simulink model "Analog_DSSS_WH"  (Simulink 7.5)
settings: Solver=ode45  SolverMode=SingleTasking  StartTime=0.0  StopTime=50  RelTol=1e-3
values from neighbouring files (symbols this model uses):
  Amp = Simulink.Parameter    [Analog_DSSS_GC_saveas.m]    (also in Analog_DSSS_WH_saveas.m)
  FreqBase = Simulink.Parameter    [Analog_DSSS_GC_saveas.m]    (also in Analog_DSSS_WH_saveas.m)
  Phs = Simulink.Parameter    [Analog_DSSS_GC_saveas.m]    (also in Analog_DSSS_WH_saveas.m)
libraries: dsparch4 x4, dspsnks4 x2
settings Model: Creator=rooki  LastModifiedBy=rooki  CovMetricSettings=dwe  CovHtmlReporting=off  covSaveCumulativeToWorkspaceVar=off  CovSaveSingleToWorkspaceVar=off  CovExternalEMLEnable=on
settings DataIOCC: LimitDataPoints=off  SaveFormat=StructureWithTime
settings OptimizationCC: ExpressionDepthLimit=128
settings DebuggingCC: UnderspecifiedInitializationDetection=Simplified  MergeDetectMultiDrivingBlocksExec=error  SolverPrmCheckMsg=none  FcnCallInpInsideContextMsg=Enable All  StateNameClashWarn=none
settings HardwareCC: ProdIntDivRoundTo=Zero  ProdEndianess=LittleEndian  ProdHWDeviceType=Specified
settings CodeAppCC: CustomSymbolStrType=$N$R$M_T
settings GRTTargetCC: TargetFunctionLibrary=C99 (ISO)  GeneratePreprocessorConditionals=Use local settings

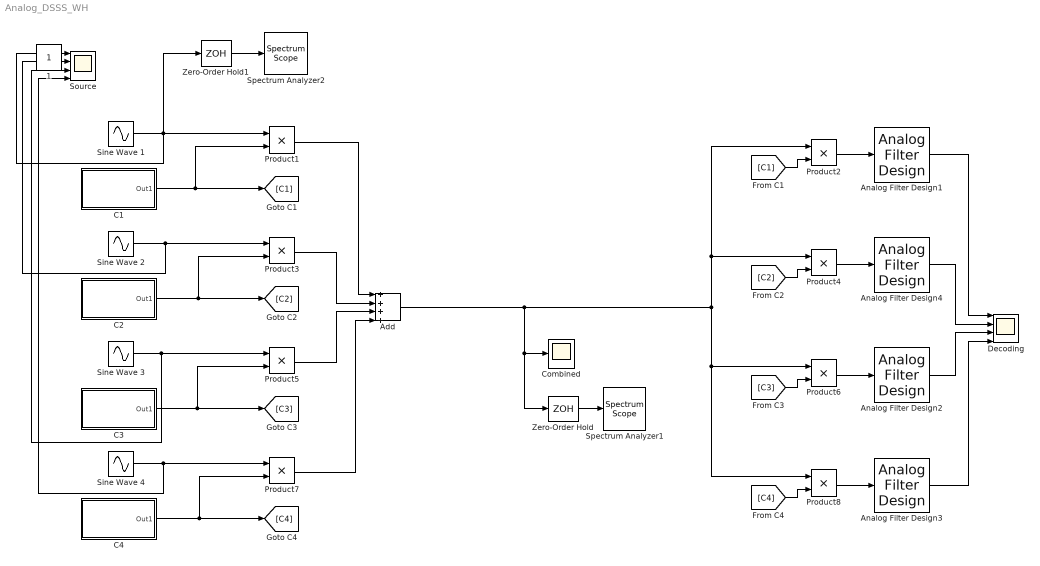
== system Analog_DSSS_WH ==
  Add : Sum  Inputs=++++
  Analog Filter Design{1..4} (4 alike) : dsparch4/Analog Filter Design  method=Butterworth  filttype=Lowpass  N=8  Wlo=2  Whi=80  Rp=2  Rs=40
  C1 : Subsystem  Description=Replaced Block
      mask Type: Replaced Block
      mask Description: This block has been replaced with an empty subsystem because it used functionality that is unavailable in Simulink R2010a.
      mask Display: fprintf('Replaced: %s\n','MATLABSystem')
  C2 : Subsystem  Description=Replaced Block
      mask Type: Replaced Block
      mask Description: This block has been replaced with an empty subsystem because it used functionality that is unavailable in Simulink R2010a.
      mask Display: fprintf('Replaced: %s\n','MATLABSystem')
  C3 : Subsystem  Description=Replaced Block
      mask Type: Replaced Block
      mask Description: This block has been replaced with an empty subsystem because it used functionality that is unavailable in Simulink R2010a.
      mask Display: fprintf('Replaced: %s\n','MATLABSystem')
  C4 : Subsystem  Description=Replaced Block
      mask Type: Replaced Block
      mask Description: This block has been replaced with an empty subsystem because it used functionality that is unavailable in Simulink R2010a.
      mask Display: fprintf('Replaced: %s\n','MATLABSystem')
  Combined : Scope
      settings: TimeRange=auto  MaxDataPoints=5000  SaveToWorkspace=off  SaveName=ScopeData2  YMin=-5.14393  YMax=5.55034  SampleTime=-1
  Decoding : Scope  NumInputPorts=4
      settings: TimeRange=auto  MaxDataPoints=5000  SaveToWorkspace=off  SaveName=ScopeData  YMin=-2.57301~-5~-5~-5  YMax=2.52348~5~5~5  SampleTime=-1
  Product{1..8} (8 alike) : Product
  Sine Wave 1 : Sin  Amplitude=Amp(1)  Frequency=FreqBase  Phase=Phs(1)  SampleTime=0
  Sine Wave 2 : Sin  Amplitude=Amp(2)  Frequency=FreqBase  Phase=Phs(2)  SampleTime=0
  Sine Wave 3 : Sin  Amplitude=Amp(3)  Frequency=FreqBase  Phase=Phs(3)  SampleTime=0
  Sine Wave 4 : Sin  Amplitude=Amp(4)  Frequency=FreqBase  Phase=Phs(4)  SampleTime=0
  Source : Scope  NumInputPorts=4
      settings: TimeRange=auto  MaxDataPoints=5000  SaveToWorkspace=off  YMin=-2.5~-5~-5~-5  YMax=2.5~5~5~5  SampleTime=-1
  Spectrum Analyzer1 : dspsnks4/Spectrum Scope  YUnits=dBm  numAvg=1  wintypeSpecScope=Hann  RsSpecScope=50  betaSpecScope=5  XRange=Two-sided  AxisGrid=on  AxisLegend=off  Memory=off  inpFftLenInherit=on  FFTlength=1024  XLimit=Auto  XMin=0  XMax=1  UseBuffer=on  BufferSize=3075  Overlap=0  FigPos="[1             41      1434.6667      847.33333]"  winsampSpecScope=Symmetric  XDisplay=0
      settings: YMin=-216.86824849143756  YMax=49.923531275391788
  Spectrum Analyzer2 : dspsnks4/Spectrum Scope  YUnits=dBm  numAvg=1  wintypeSpecScope=Hann  RsSpecScope=50  betaSpecScope=5  XRange=Two-sided  AxisGrid=on  AxisLegend=off  Memory=off  inpFftLenInherit=on  FFTlength=1024  XLimit=User-defined  XMin=-1  XMax=1  UseBuffer=on  BufferSize=3075  Overlap=0  FigPos="[1             41      1434.6667      847.33333]"  winsampSpecScope=Symmetric  XDisplay=0
      settings: YMin=-216.86824849143756  YMax=49.923531275391788
  Zero-Order Hold : ZeroOrderHold  SampleTime=1/32
  Zero-Order Hold1 : ZeroOrderHold  SampleTime=1/32
  1 : Constant  IOType=siggen
  wires:
  C1/1(Out1) -> Product1/2, [C1]
  Zero-Order Hold/1 -> Spectrum Analyzer1/1
  C2/1(Out1) -> [C2], Product3/2
  Product1/1 -> Add/1
  Product3/1 -> Add/2
  Product2/1 -> Analog Filter Design1/1
  Analog Filter Design1/1 -> Decoding/1
  Product5/1 -> Add/3
  C3/1(Out1) -> [C3], Product5/2
  Add/1 -> Zero-Order Hold/1, Combined/1, Product8/1, Product6/1, Product4/1, Product2/1
  Product7/1 -> Add/4
  C4/1(Out1) -> [C4], Product7/2
  Sine Wave 2/1 -> Source/2, Product3/1
  Sine Wave 3/1 -> Source/3, Product5/1
  Sine Wave 4/1 -> Source/4, Product7/1
  [C1] -> Product2/2
  [C2] -> Product4/2
  Product4/1 -> Analog Filter Design4/1
  Product6/1 -> Analog Filter Design2/1
  [C3] -> Product6/2
  Product8/1 -> Analog Filter Design3/1
  [C4] -> Product8/2
  Analog Filter Design4/1 -> Decoding/2
  Analog Filter Design2/1 -> Decoding/3
  Analog Filter Design3/1 -> Decoding/4
  Zero-Order Hold1/1 -> Spectrum Analyzer2/1
  Sine Wave 1/1 -> Zero-Order Hold1/1, Source/1, Product1/1

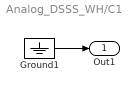
== system Analog_DSSS_WH/C1 ==
  Ground1 : Ground
  Out1 : Outport
  wires:
  Ground1/1 -> Out1/1

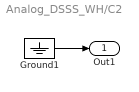
== system Analog_DSSS_WH/C2 ==
  Ground1 : Ground
  Out1 : Outport
  wires:
  Ground1/1 -> Out1/1

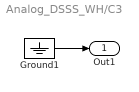
== system Analog_DSSS_WH/C3 ==
  Ground1 : Ground
  Out1 : Outport
  wires:
  Ground1/1 -> Out1/1

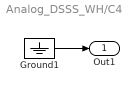
== system Analog_DSSS_WH/C4 ==
  Ground1 : Ground
  Out1 : Outport
  wires:
  Ground1/1 -> Out1/1
